simulink model "DenseThinHyst"  (R2025a)
settings: Solver=FixedStepDiscrete  StartTime=0.0  StopTime=10.0  FixedStep=0.1  RelTol=1e-3
settings Model: Creator=dinhnamnguyen  LastModifiedBy=dinhnamnguyen

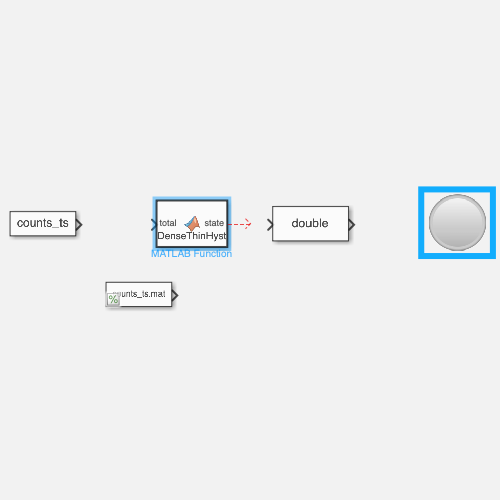
[thumbnail: Simulink's stored preview of the top-level diagram]
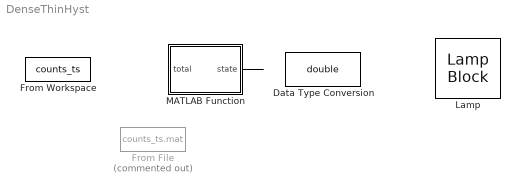
== system DenseThinHyst ==
  Data Type Conversion : DataTypeConversion  OutDataTypeStr=double  SaturateOnIntegerOverflow=off  RndMeth=Floor
  From Workspace : FromWorkspace  VariableName=counts_ts  SampleTime=-1
  From File : FromFile  Commented=on  FileName=counts_ts.mat
  Lamp : LampBlock  LabelPosition=Hide  DefaultColor=[192.0, 192.0, 192.0]
  MATLAB Function : MATLAB Function  TreatAsAtomicUnit=on
  wires:
  MATLAB Function/1(state) -> ?

== matlab function DenseThinHyst/MATLAB Function ==
  data: total input; state output
function state = DenseThinHyst(total)
% Returns 0/1 (double) directly for Lamp
% total: scalar double (total vehicles at current step)
%
% Tunables (adjust to your data & model step):
TH_DENSE   = 10;   % >=10 -> dense
TH_THIN    = 3;    % <=3  -> thin
HOLD_TICKS = 10;   % number of MODEL STEPS to wait before switching
                   % e.g., if step = 0.1 s, 10 ticks ≈ 1.0 s

%#codegen
persistent s cnt
if isempty(s)
    s   = uint8(0);   % 0=thin, 1=dense
    cnt = uint16(0);
end

% Decide desired state by thresholds (no ROI, total-only)
desired = s;
if total >= TH_DENSE
    desired = uint8(1);
elseif total <= TH_THIN
    desired = uint8(0);
end

% Hysteresis by holding for HOLD_TICKS samples
if desired ~= s
    cnt = cnt + 1;
    if cnt >= uint16(HOLD_TICKS)
        s = desired;
        cnt = uint16(0);
    end
else
    cnt = uint16(0);
end

% Output as numeric 0/1 (double) for Lamp
state = double(s);
